simulink model "svpwm"  (R2026a)
settings: Solver=VariableStepAuto
libraries: mcbeeMathTransformLib x2, eePwmGeneratorTwoLevel x1

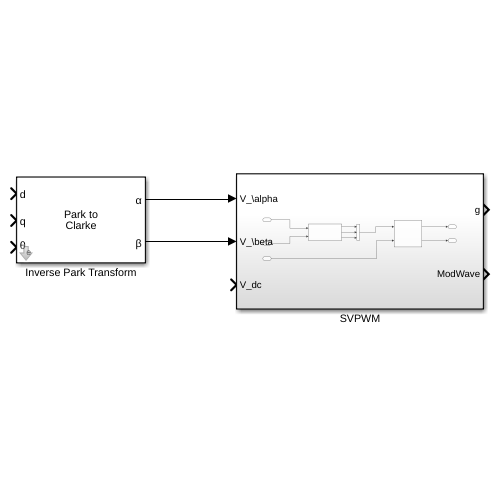
[thumbnail: Simulink's stored preview of the top-level diagram]
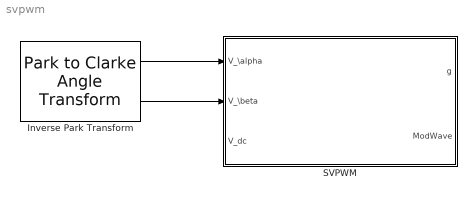
== system svpwm ==
  Inverse Park Transform : mcbeeMathTransformLib/Park to Clarke Angle Transform  AxisAlignment=D-axis  UseWithEmbedded=on  PhaseInput=Two inputs  ThetaInput=Electrical position  AngleInput=Radians  N_points=1024
      settings: LibrarySourceBlock=mcbhdllib/Controls/Math Transforms/Inverse Park Transform
  SVPWM : Subsystem
  wires:
  Inverse Park Transform/1 -> SVPWM/1(V_\alpha)
  Inverse Park Transform/2 -> SVPWM/2(V_\beta)

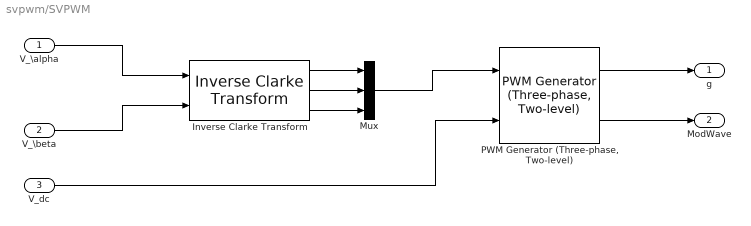
== system svpwm/SVPWM ==
  V_\alpha : Inport
  V_\beta : Inport  Port=2
  V_dc : Inport  Port=3
  Inverse Clarke Transform : mcbeeMathTransformLib/Inverse Clarke Transform  PowerInvariant=off  UseWithEmbedded=on  PhaseInput=Two inputs
      settings: LibrarySourceBlock=mcbhdllib/Controls/Math Transforms/Inverse Clarke Transform
  Mux : Mux  Inputs=3
  "PWM Generator (Three-phase, Two-level)" : eePwmGeneratorTwoLevel/PWM Generator (Three-phase, Two-level)  PWMMode=Continuous PWM (CPWM)  CPWMMode=SVM: space vector modulation  DPWMMode=60 DPWM: 60 degree discontinuous PWM  fsw=1e3  Ts=5e-5
      settings: LibrarySourceBlock=|
      | ee_sl_lib/Pulse Width
      | Modulation/PWM Generator
      | (Three-phase, Two-level)
  g : Outport
  ModWave : Outport  Port=2
  wires:
  V_\alpha/1 -> Inverse Clarke Transform/1
  V_\beta/1 -> Inverse Clarke Transform/2
  Inverse Clarke Transform/1 -> Mux/1
  Inverse Clarke Transform/2 -> Mux/2
  Inverse Clarke Transform/3 -> Mux/3
  Mux/1 -> "PWM Generator (Three-phase, Two-level)"/1
  "PWM Generator (Three-phase, Two-level)"/1 -> g/1
  "PWM Generator (Three-phase, Two-level)"/2 -> ModWave/1
  V_dc/1 -> "PWM Generator (Three-phase, Two-level)"/2
